simulink model "Safety_filter_obstacle_run_FxTISMC"  (R2022a)
settings: Solver=ode4  StartTime=0.0  StopTime=30  FixedStep=0.01  RelTol=1e-3
libraries: simulink x1
settings Model: PacingRate=0.500000  Creator=14244039  LastModifiedBy=40335991
settings DebuggingCC: UnconnectedInputMsg=warning  UnconnectedOutputMsg=warning  UnconnectedLineMsg=warning  UnderSpecifiedDimensionMsg=warning
settings RTWCC: DLArmComputeVersion=19.05

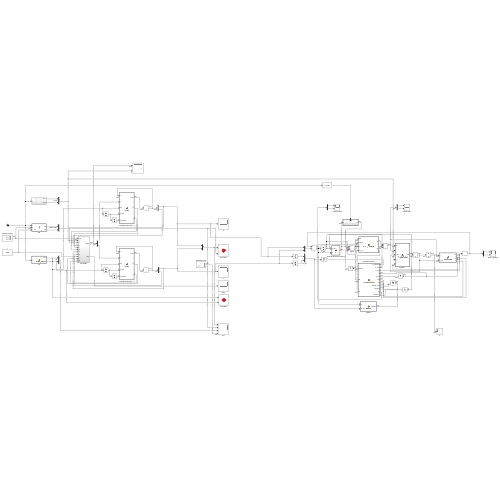
[thumbnail: Simulink's stored preview of the top-level diagram]
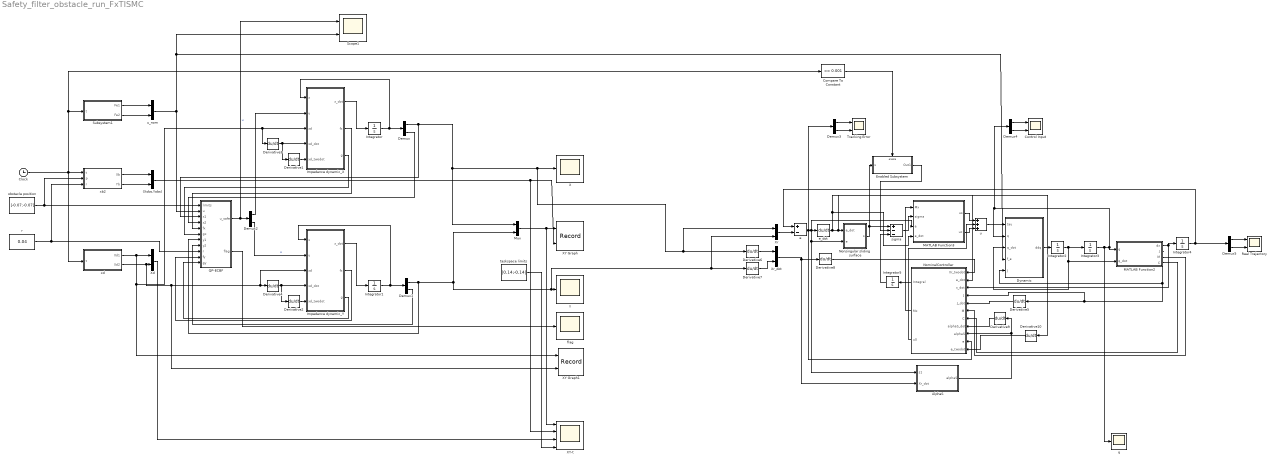
== system Safety_filter_obstacle_run_FxTISMC ==
  " Tracking Error" : Scope  NumInputPorts=2
  (Xobs,Yobs) : Mux  Inputs=2
  AlphaS : MATLAB Function  TreatAsAtomicUnit=on
  Clock : Clock
  Compare To Constant : simulink/Logic and Bit Operations/Compare To Constant  relop=<=  const=0.001  OutDataTypeStr=boolean
  Control Input : Scope  NumInputPorts=2
  Demux{,1..5} (6 alike) : Demux  Outputs=2
  Derivative{1..10} (10 alike) : Derivative
  Dynamic : MATLAB Function  TreatAsAtomicUnit=on
  Enabled Subsystem : Subsystem  TreatAsAtomicUnit=on
  Impedance dynamic_X : MATLAB Function  TreatAsAtomicUnit=on
  Impedance dynamic_Y : MATLAB Function  TreatAsAtomicUnit=on
  Integrator : Integrator  InitialCondition=[0.14;0]
  Integrator1 : Integrator  InitialCondition=[0;0]
  Integrator2 : Integrator
  Integrator3 : Integrator  InitialCondition=[0.5236;2.0944]
  Integrator4 : Integrator  InitialCondition=[0.14;0]
  Integrator5 : Integrator  InitialCondition=[0.0001;0.0001]
  MATLAB Function2 : MATLAB Function  TreatAsAtomicUnit=on
  MATLAB Function3 : MATLAB Function  TreatAsAtomicUnit=on
  Mux : Mux  Inputs=2
  NominalController : MATLAB Function  TreatAsAtomicUnit=on
  Nonsingular sliding surface : MATLAB Function  TreatAsAtomicUnit=on
  QP-ECBF : Subsystem
  Real Trajectory : Scope  NumInputPorts=2
  Scope1 : Scope  NumInputPorts=2
  Subsystem1 : Subsystem
  X : Scope
  XY Graph : Record  FileSettingsInternal="{\"entries\":[{\"content\":{\"excelSettings\":{\"content\":{},\"type\":\"Streamout.ExcelSettings\"}},\"type\":\"Streamout.FileSettingStorage\",\"uuid\":\"41ee0d73-6c9a-4a32-9ae2-bb77aa5eb9da\"}],\"packageUris\":[\"http://schema.mathworks.com/mf0/streamout_blocks/R2020a\"],\"version\":\"1.0\"}"  Layout=[1 1]  SignalsInternal="{\"entries\":[{\"content\":{\"signals\":[{\"content\":{\"blockPath\":[\"Safety_filter_obstacle_run_FxTISMC/XY Graph\"],\"channel\":[],\"dimensions\":[2],\"domain\":\"Safety_filter_obstacle_run_FxTISMC/XY Graph\",\"hasChildren\":true,\"lineColor\":\"#0072bd\",\"plots\":[],\"port\":1,\"sid\":[\"\"],\"signalID\":13917,\"signalName\":\"Mux\"},\"type\":\"RecordBlkView.Signal\",\"uuid\":\"9d963ae4-670a-439a-a92f-b214391dedbc\"},{\"content\":{\"blockPath\":[\"Safety_filter_obstacle_run_FxTISMC/XY Graph\"],\"channel\":[1],\"dimensions\":[2],\"domain\":\"Safety_filter_obstacle_run_FxTISMC/XY Graph\",\"lineColor\":\"#d95319\",\"parentID\":13917,\"plots\":[1],\"port\":1,\"sid\":[\"\"],\"signalID\":13918,\"signalName\":\"Mux\"},\"type\":\"RecordBlkView.Signal\",\"uuid\":\"5de3c74c-0cc7-4e71-b0b3-a53949196780\"},{\"content\":{\"blockPath\":[\"Safety_filter_obstacle_run_FxTISMC/XY Graph\"],\"channel\":[],\"dimensions\":[2],\"domain\":\"Safety_filter_obstacle_run_FxTISMC/XY Graph\",\"hasChildren\":true,\"lineColor\":\"#edb120\",\"plots\":[],\"port\":2,\"sid\":[\"\"],\"signalID\":13922,\"signalName\":\"(Xobs,Yobs)\"},\"type\":\"RecordBlkView.Signal\",\"uuid\":\"3f86d34b-246c-421d-b9f1-6aa0b0fd2e9d\"},{\"content\":{\"blockPath\":[\"Safety_filter_obstacle_run_FxTISMC/XY Graph\"],\"channel\":[1],\"dimensions\":[2],\"domain\":\"Safety_filter_obstacle_run_FxTISMC/XY Graph\",\"lineColor\":\"#7e2f8e\",\"parentID\":13922,\"plots\":[1],\"port\":2,\"sid\":[\"\"],\"signalID\":13923,\"signalName\":\"(Xobs,Yobs)\"},\"type\":\"RecordBlkView.Signal\",\"uuid\":\"b5bee711-287f-47f0-862a-4f60470f5475\"},{\"content\":{\"blockPath\":[\"Safety_filter_obstacle_run_FxTISMC/XY Graph\"],\"channel\":[2],\"dimensions\":[2],\"domain\":\"Safety_filter_obstacle_run_FxTISMC/XY Graph\",\"lineColor\":\"#a2142f\",\"parentID\":13917,\"plots\":[1],\"port\":1,\"sid\":[\"\"],\"signalID\":13935,\"signalName\":\"Mux\"},\"type\":\"RecordBlkView.Signal\",\"uuid\":\"9dfeebbb-1213-4c0a-aa59-e1486d2e2cfe\"},{\"content\":{\"blockPath\":[\"Safety_filter_obstacle_run_FxTISMC/XY Graph\"],\"channel\":[2],\"dimensions\":[2],\"domain\":\"Safety_filter_obstacle_run_FxTISMC/XY Graph\",\"lineColor\":\"#139fff\",\"parentID\":13922,\"plots\":[1],\"port\":2,\"sid\":[\"\"],\"signalID\":13936,\"signalName\":\"(Xobs,Yobs)\"},\"type\":\"RecordBlkView.Signal\",\"uuid\":\"a1ac44f8-5473-466a-96b0-ad1e605dc7af\"}]},\"type\":\"RecordBlkView.InputSignals\",\"uuid\":\"7214ea23-0c5e-4860-8b5d-1e1159aeb053\"}],\"packageUris\":[\"http://schema.mathworks.com/mf0/streamout_blocks/R2020a\"],\"version\":\"1.0\"}"  VisualizationBindings="{\"xyplotplugin\":{\"info\":[{\"series\":[{\"bindingParametersList\":[{\"parameter\":\"X-Axis\",\"signalID\":13918,\"signalName\":\"Mux(1)\"},{\"parameter\":\"Y-Axis\",\"signalID\":13935,\"signalName\":\"Mux(2)\"}],\"seriesID\":62594},{\"bindingParametersList\":[{\"parameter\":\"X-Axis\",\"signalID\":13923,\"signalName\":\"(Xobs,Yobs)(1)\"},{\"parameter\":\"Y-Axis\",\"signalID\":13936,\"signalName\":\"(Xobs,Yobs)(2)\"}],\"seriesID\":13492}],\"subplotID\":1}]}}"  CompatibilityTag=XY  st=-1
  XY Graph1 : Record  FileSettingsInternal="{\"entries\":[{\"content\":{\"excelSettings\":{\"content\":{},\"type\":\"Streamout.ExcelSettings\"}},\"type\":\"Streamout.FileSettingStorage\",\"uuid\":\"947f9a06-cda0-4a39-953d-72ad5f3dd9f2\"}],\"packageUris\":[\"http://schema.mathworks.com/mf0/streamout_blocks/R2020a\"],\"version\":\"1.0\"}"  Layout=[1 1]  SignalsInternal="{\"entries\":[{\"content\":{\"signals\":[{\"content\":{\"blockPath\":[\"Safety_filter_obstacle_run_FxTISMC/XY Graph1\"],\"channel\":[],\"dimensions\":[1],\"domain\":\"Safety_filter_obstacle_run_FxTISMC/XY Graph1\",\"lineColor\":\"#a2142f\",\"plots\":[1],\"port\":1,\"sid\":[\"\"],\"signalID\":13927,\"signalName\":\"xd:1\"},\"type\":\"RecordBlkView.Signal\",\"uuid\":\"bb191c1c-9b05-4e6a-a985-f226d7343dd8\"},{\"content\":{\"blockPath\":[\"Safety_filter_obstacle_run_FxTISMC/XY Graph1\"],\"channel\":[],\"dimensions\":[1],\"domain\":\"Safety_filter_obstacle_run_FxTISMC/XY Graph1\",\"lineColor\":\"#139fff\",\"plots\":[1],\"port\":2,\"sid\":[\"\"],\"signalID\":13931,\"signalName\":\"xd:2\"},\"type\":\"RecordBlkView.Signal\",\"uuid\":\"5ec12a56-9b42-4693-a6cf-ba7cb0d2111f\"}]},\"type\":\"RecordBlkView.InputSignals\",\"uuid\":\"53783b2f-f43d-4ce0-a107-2c856c2899e0\"}],\"packageUris\":[\"http://schema.mathworks.com/mf0/streamout_blocks/R2020a\"],\"version\":\"1.0\"}"  VisualizationBindings="{\"xyplotplugin\":{\"info\":[{\"series\":[{\"bindingParametersList\":[{\"parameter\":\"X-Axis\",\"signalID\":13927,\"signalName\":\"xd:1\"},{\"parameter\":\"Y-Axis\",\"signalID\":13931,\"signalName\":\"xd:2\"}],\"seriesID\":52353}],\"subplotID\":1}]}}"  CompatibilityTag=XY
  XY-t : Scope  NumInputPorts=4
  Xd : Mux  Inputs=2
  Xr : Mux  Inputs=2
  Xr_dot : Mux  Inputs=2
  Y : Scope
  e : Sum  Inputs=+-
  e_dot : Derivative
  flag : Scope
  obstacle position : Constant  Value=[-0.07;-0.07]  VectorParams1D=off  SampleTime=-1
  q : Scope
  r : Constant  Value=0.04  VectorParams1D=off  SampleTime=-1
  sigma : Sum  Inputs=+--
  taskspace limits : Constant  Value=[0.14;-0.14]  VectorParams1D=off  SampleTime=-1
  u : Sum  Inputs=+++
  u_nom : Mux  Inputs=2
  xb2 : MATLAB Function  TreatAsAtomicUnit=on
  xd : MATLAB Function  TreatAsAtomicUnit=on
  wires:
  Subsystem1/1(Fe1) -> u_nom/1
  Clock/1 -> Compare To Constant/1, Subsystem1/1(t), xd/1(t), xb2/1(t)
  Derivative3/1 -> Impedance dynamic_X/4(xd_dot), Derivative1/1
  Derivative1/1 -> Impedance dynamic_X/5(xd_twodot)
  Impedance dynamic_X/1(x_dot) -> Integrator/1
  Integrator/1 -> Demux/1, Impedance dynamic_X/1(x)
  Demux2/2 -> Impedance dynamic_Y/2(u)  "u"
  xd/2(Xd2) -> XY Graph1/2, Impedance dynamic_Y/3(xd), Derivative4/1, Xd/2
  Impedance dynamic_Y/1(x_dot) -> Integrator1/1
  Derivative4/1 -> Impedance dynamic_Y/4(xd_dot), Derivative2/1
  Derivative2/1 -> Impedance dynamic_Y/5(xd_twodot)
  Integrator1/1 -> Demux1/1, Impedance dynamic_Y/1(x)
  Subsystem1/2(Fe2) -> u_nom/2
  xb2/1(Xb) -> (Xobs,Yobs)/1
  xb2/2(Yb) -> (Xobs,Yobs)/2
  Mux/1 -> XY-t/1, XY Graph/1
  (Xobs,Yobs)/1 -> XY-t/2, XY Graph/2
  QP-ECBF/1(u_safe) -> Scope1/1, Demux2/1  "u"
  Demux2/1 -> Impedance dynamic_X/2(u)
  obstacle position/1 -> QP-ECBF/1(limits), xb2/2(p)
  Demux/2 -> QP-ECBF/4(x2)
  Impedance dynamic_X/2(fx) -> QP-ECBF/5(fx)
  Impedance dynamic_X/3(g) -> QP-ECBF/6(gx)
  Demux1/2 -> QP-ECBF/8(y2)
  r/1 -> xb2/3(r), QP-ECBF/9(r)
  QP-ECBF/2(flag) -> flag/1
  Impedance dynamic_Y/2(fx) -> QP-ECBF/10(fy)
  Impedance dynamic_Y/3(g) -> QP-ECBF/11(gy)
  xd/1(Xd1) -> XY Graph1/1, Impedance dynamic_X/3(xd), Derivative3/1, Xd/1
  Xd/1 -> XY-t/3
  taskspace limits/1 -> XY-t/4
  NominalController/1(Integral) -> Integrator5/1
  Demux5/2 -> Real Trajectory/2
  Demux4/2 -> Control Input/2
  Integrator5/1 -> sigma/3
  u_nom/1 -> Dynamic/4(f_e), Scope1/2, QP-ECBF/2(u)
  e_dot/1 -> MATLAB Function3/4(e_dot), Derivative10/1, NominalController/2(e_dot), Nonsingular sliding surface/1(e_dot)
  Nonsingular sliding surface/1(s) -> Enabled Subsystem/1(s), sigma/1
  Demux4/1 -> Control Input/1
  AlphaS/1(alphaS) -> Derivative9/1, NominalController/9(alphaS)
  Enabled Subsystem/1(Out1) -> sigma/2
  Demux3/2 -> " Tracking Error"/2
  Dynamic/1(ddq) -> Integrator2/1
  Demux3/1 -> " Tracking Error"/1
  Xr/1 -> e/2
  Compare To Constant/1 -> Enabled Subsystem/Enable
  MATLAB Function2/4(C) -> NominalController/7(C)
  Derivative9/1 -> NominalController/8(alphaS_dot)
  MATLAB Function3/1(us) -> u/1
  MATLAB Function2/1(dx) -> Integrator4/1, NominalController/3(x_dot)
  MATLAB Function3/2(uc) -> u/3
  Derivative10/1 -> NominalController/11(e_twodot)
  Derivative8/1 -> NominalController/1(Xr_twodot)
  u/1 -> Dynamic/1(tau)
  MATLAB Function2/2(J) -> Dynamic/5(J), NominalController/4(J), Derivative5/1
  Integrator3/1 -> q/1, Demux4/1, Dynamic/2(q), MATLAB Function2/1(q)
  Xr_dot/1 -> AlphaS/2(Xr_dot), Derivative8/1
  sigma/1 -> MATLAB Function3/2(sigma)
  Integrator4/1 -> Demux5/1, e/1
  MATLAB Function2/3(M) -> NominalController/6(M)
  e/1 -> Demux3/1, e_dot/1, MATLAB Function3/3(e), AlphaS/1(s1), Nonsingular sliding surface/2(e), NominalController/10(e)
  NominalController/2(Mx) -> MATLAB Function3/1(Mx)
  Integrator2/1 -> MATLAB Function2/2(q_dot), Dynamic/3(q_dot), Integrator3/1
  NominalController/3(u0) -> u/2
  Demux5/1 -> Real Trajectory/1
  Derivative5/1 -> NominalController/5(J_dot)
  Demux1/1 -> QP-ECBF/7(y1), Xr/2, Derivative7/1, Y/1, Mux/2
  Demux/1 -> QP-ECBF/3(x1), Mux/1, Xr/1, Derivative6/1, X/1
  Derivative6/1 -> Xr_dot/1
  Derivative7/1 -> Xr_dot/2

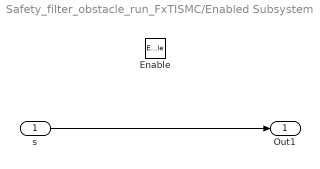
== system Safety_filter_obstacle_run_FxTISMC/Enabled Subsystem ==
  s : Inport
  Enable : EnablePort
  Out1 : Outport  InitialOutput=0  VectorParamsAs1DForOutWhenUnconnected=off
  wires:
  s/1 -> Out1/1

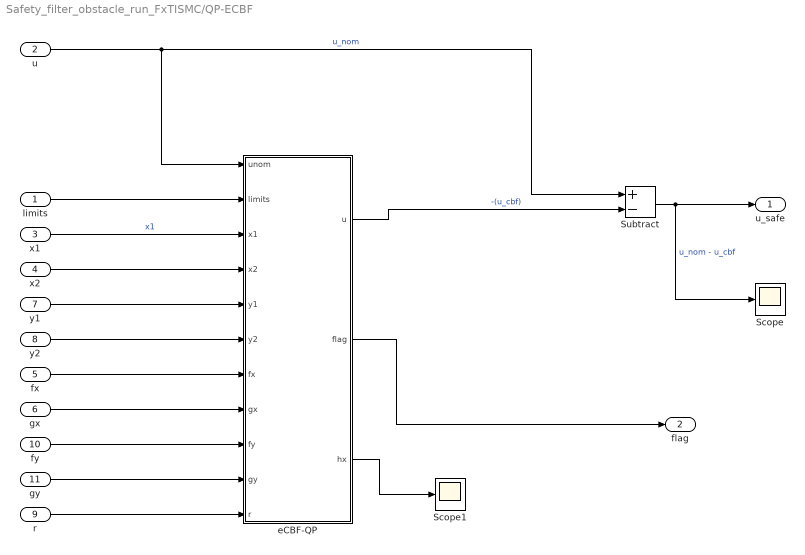
== system Safety_filter_obstacle_run_FxTISMC/QP-ECBF ==
  limits : Inport
  u : Inport  Port=2
  x1 : Inport  Port=3
  x2 : Inport  Port=4
  fx : Inport  Port=5
  gx : Inport  Port=6
  y1 : Inport  Port=7
  y2 : Inport  Port=8
  r : Inport  Port=9
  fy : Inport  Port=10
  gy : Inport  Port=11
  Scope : Scope
  Scope1 : Scope
  Subtract : Sum  Inputs=+-
  eCBF-QP : MATLAB Function  TreatAsAtomicUnit=on
  u_safe : Outport
  flag : Outport  Port=2
  wires:
  x2/1 -> eCBF-QP/4(x2)
  limits/1 -> eCBF-QP/2(limits)
  u/1 -> eCBF-QP/1(unom), Subtract/1  "u_nom"
  x1/1 -> eCBF-QP/3(x1)  "x1"
  eCBF-QP/1(u) -> Subtract/2  "-(u_cbf)"
  Subtract/1 -> u_safe/1, Scope/1  "u_nom - u_cbf"
  fx/1 -> eCBF-QP/7(fx)
  gx/1 -> eCBF-QP/8(gx)
  eCBF-QP/2(flag) -> flag/1
  y1/1 -> eCBF-QP/5(y1)
  y2/1 -> eCBF-QP/6(y2)
  r/1 -> eCBF-QP/11(r)
  eCBF-QP/3(hx) -> Scope1/1
  fy/1 -> eCBF-QP/9(fy)
  gy/1 -> eCBF-QP/10(gy)

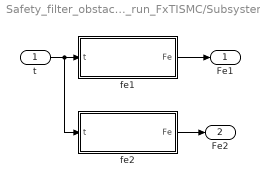
== system Safety_filter_obstacle_run_FxTISMC/Subsystem1 ==
  t : Inport
  fe1 : MATLAB Function  TreatAsAtomicUnit=on
  fe2 : MATLAB Function  TreatAsAtomicUnit=on
  Fe1 : Outport
  Fe2 : Outport  Port=2
  wires:
  fe1/1(Fe) -> Fe1/1
  fe2/1(Fe) -> Fe2/1
  t/1 -> fe2/1(t), fe1/1(t)

== matlab function Safety_filter_obstacle_run_FxTISMC/MATLAB Function2 ==
  data: q input; q_dot input; dx output; J output; M output; C output
function [dx,J,M,C]  = JointTwoTask(q,q_dot)
L = [0.3, 0.3];
m = [1.5, 1];

M = [m(2)*L(2)^2+2*m(2)*L(1)*L(2)*cos(q(2))+(m(1)+m(2))*L(1)^2, m(2)*L(2)^2+m(2)*L(1)*L(2)*cos(q(2));
    m(2)*L(2)^2+m(2)*L(1)*L(2)*cos(q(2)), m(2)*L(2)^2];
C = [-2*m(2)*L(1)*L(2)*sin(q(2))*q_dot(2), -m(2)*L(1)*L(2)*sin(q(2)); 
    m(2)*L(1)*L(2)*sin(q(2))*q_dot(1), 0];
J = [-L(1)*sin(q(1))-L(2)*sin(q(1)+q(2)), -L(2)*sin(q(1)+q(2));
    L(1)*cos(q(1))+L(2)*cos(q(1)+q(2)), L(2)*cos(q(1)+q(2))];
dx = J*q_dot;
end

== matlab function Safety_filter_obstacle_run_FxTISMC/AlphaS ==
  data: s1 input; alphaS output; Xr_dot input
function alphaS = AlphaS(s1,Xr_dot)

k1=3;
k2=20;
k3=50;

alpha=5/7;
beta=5/3;

alphaS = -(k1.*s1 + k2.*abs(s1).^alpha.*sign(s1) + k3.*abs(s1).^beta.*sign(s1)) + Xr_dot;

end

== matlab function Safety_filter_obstacle_run_FxTISMC/MATLAB Function3 ==
  data: Mx input; us output; sigma input; uc output; e input; e_dot input
function [us,uc] = ISMC_Controller(Mx,sigma,e,e_dot)

K_gain=0.001;
k1=20;
k2=50;
alpha=5/3;
beta=5/7;
Mxx=pinv(Mx);
gamma = 5/7;
us = -inv(Mx)*((K_gain+0.001)*sign(sigma) + k1*abs(sigma).^alpha.*sign(sigma) + k2*abs(sigma).^beta.*sign(sigma));
% uc = -Mxx*k2^gamma*(abs(e_dot+k1*abs(e).^alpha.*sign(e)).^(1/gamma-1)).*e_dot;
uc = 0;
end

== matlab function Safety_filter_obstacle_run_FxTISMC/NominalController ==
  data: Xr_twodot input; e_dot input; x_dot input size=[2 1]; J input; J_dot input; M input; C input; alphaS_dot input size=[2 1]; Integral output size=[2 1]; Mx output size=[2 2]; u0 output size=[2 1]; alphaS input; e input; e_twodot input
function [Integral,Mx,u0] = NominalController(Xr_twodot,e_dot,x_dot,J,J_dot,M,C,alphaS_dot,alphaS,e,e_twodot)

Mx = inv(J')*M*inv(J);
Cx = inv(J')*(C-(M*inv(J)*J_dot))*inv(J);

%% PD Controller
% Kp=35;
% Kd=400;
% f=Mx*(Kp*(Xr-x)+Kd*(Xr_dot-x_dot)) + Cx*x_dot;
% u0=(J')*f;

%% Fixed-time backstepping control
k8=3;
k9=20;
k10=50;
alpha=5/3;
beta=5/7;
gamma = 5/7;

s2 = x_dot - alphaS;

f0 = Mx*(inv(Mx)*Cx*x_dot + alphaS_dot - k8*s2 - k9*abs(s2).^alpha.*sign(s2) - k10*abs(s2).^beta.*sign(s2));
u0=(J')*f0;

%% Integral term of fixed-time integral sliding mode controller

k1=20;
k2=50;
%  Integral = Mx\u0 +  Mx\Cx*x_dot - Xr_twodot + e_dot + (1/k2^gamma)*(abs(e_dot+k1*abs(e).^alpha.*sign(e)).^(1/gamma-1)).*(Mx\u0 +  Mx\Cx*x_dot - Xr_twodot + k1*abs(e).^(alpha-1).*e_dot);
Integral = e_dot + (1/k2^gamma)*(abs(e_dot+k1*abs(e).^alpha.*sign(e)).^(1/gamma-1)).*(Mx\u0 +  Mx\Cx*x_dot - Xr_twodot + k1*abs(e).^(alpha-1).*e_dot);


end

== matlab function Safety_filter_obstacle_run_FxTISMC/Nonsingular sliding surface ==
  data: e_dot input; e input; s output
function s = S(e_dot,e)

k1=20;
k2=50;
alpha=5/3;
beta=5/7;
gamma = 5/7;

s = e + (1/k2^(gamma)).*abs(e_dot+k1*abs(e).^alpha.*sign(e)).^(1/gamma).*sign(e_dot+k1*abs(e).^alpha.*sign(e));

end

== matlab function Safety_filter_obstacle_run_FxTISMC/xb2 ==
  data: t input; Xb output; Yb output; p input; r input
function [Xb,Yb]  = Obstacles_traj(t,p,r)

Xb =  p(1) + r*cos(t);
Yb =  p(2) + r*sin(t);
    
end

== matlab function Safety_filter_obstacle_run_FxTISMC/Impedance dynamic_Y ==
  data: x input size=[2 1]; u input; x_dot output size=[2 1]; xd input; xd_dot input; xd_twodot input; fx output; g output
function [x_dot,fx,g] = System(x,u,xd,xd_dot,xd_twodot)

    km = 20;
    kb = 20;                                                       
    kk = 100;
    fx = [x(2);
        -(1/km)*(kb*(x(2)-xd_dot)+kk*(x(1)-xd)-km*xd_twodot)];
    g = [0;km^(-1)];
    x_dot = fx + g*u;
end

== matlab function Safety_filter_obstacle_run_FxTISMC/Subsystem1/fe1 ==
  data: t input; Fe output
function Fe  = External_force(t)

   Fe = 0*(t<4|t>=11) + (1-cos(pi*t))*(t>=4&t<5) + 2*(t>=5&t<10) + (1+cos(pi*t))*(t>=10&t<11);

end

== matlab function Safety_filter_obstacle_run_FxTISMC/Dynamic ==
  data: tau input size=[2 1]; ddq output size=[2 1]; q input size=[2 1]; q_dot input size=[2 1]; f_e input; J input
function ddq  = TwoLinkRobot(tau,q,q_dot,f_e,J)
L = [0.3, 0.3];
m = [1.5, 1];
g = 9.8;

M = [m(2)*L(2)^2+2*m(2)*L(1)*L(2)*cos(q(2))+(m(1)+m(2))*L(1)^2, m(2)*L(2)^2+m(2)*L(1)*L(2)*cos(q(2));
    m(2)*L(2)^2+m(2)*L(1)*L(2)*cos(q(2)), m(2)*L(2)^2];
C = [-2*m(2)*L(1)*L(2)*sin(q(2))*q_dot(2), -m(2)*L(1)*L(2)*sin(q(2)); 
    m(2)*L(1)*L(2)*sin(q(2))*q_dot(1), 0];

F=[2*cos(q(1))*sin(q(2))+5*cos(q(1))^2;-2*cos(q(1))*sin(q(2))-5*cos(q(1))^2];

tau_e = (J')*f_e;
ddq = M\(-C*q_dot-F + tau + tau_e);

end

== matlab function Safety_filter_obstacle_run_FxTISMC/Subsystem1/fe2 ==
  data: t input; Fe output
function Fe  = External_force(t)

   Fe = 0*(t<4|t>=11) + 2*(1-cos(pi*t))*(t>=4&t<5) + 4*(t>=5&t<10) + 2*(1+cos(pi*t))*(t>=10&t<11);

end

== matlab function Safety_filter_obstacle_run_FxTISMC/xd ==
  data: t input; Xd1 output; Xd2 output
function [Xd1, Xd2] = Desired_traj(t)

    Xd1=0.14*cos(0.5*t);
    Xd2=0.14*sin(0.5*t);
    
end

== matlab function Safety_filter_obstacle_run_FxTISMC/QP-ECBF/eCBF-QP ==
  settings: updateMethod=DISCRETE
  data: unom input; limits input; u output size=[2 1]; x1 input; x2 input; y1 input; y2 input; fx input; gx input; fy input; gy input; flag output; r input; hx output
function [u,flag,hx] = fcn(unom, limits, x1, x2,y1 ,y2 ,fx,gx,fy,gy,r)
    %% Obstacle position
    X_obs    = limits(1);
    Y_obs    = limits(2);
    fe_x = unom(1);
    fe_y = unom(2);
    %% ECBF Gains
    k1 = 70;
    k2 = 700;
    r = r+0.01;
    %% CBF 
    hx      = (x1 - X_obs)^2 + (y1 - Y_obs)^2 - r^2 ; 
    Lfhx    = 2*(x1 - X_obs)*x2 + 2*(y1 - Y_obs)*y2;
    L2fhx_unom = 2*(x1 - X_obs)*( gx(2)*fe_x) + 2*(y1 - Y_obs)*( gy(2)*fe_y) ;

    L2fhx_usafe_x = 2*(x1 - X_obs)*gx(2);
    L2fhx_usafe_y = 2*(y1 - Y_obs)*gy(2);
   

    H       = [2 0; 0 2];
    f       = [0;0]; 
    
    A       = [L2fhx_usafe_x, L2fhx_usafe_y]; 
            
    b       = [L2fhx_unom + k1*Lfhx + k2*hx];
    X   = [0;0];
    flag = 0;
    coder.extrinsic('quadprog');
    [output, ~, flag]   = quadprog(H,f,A,b,[],[],[],[]);

    if flag == 1
        X = output;
    else
        X   = [0;0];
    end
    
%Function outputs
    u = X; 
end

== matlab function Safety_filter_obstacle_run_FxTISMC/Impedance dynamic_X ==
  data: x input size=[2 1]; u input; x_dot output size=[2 1]; xd input; xd_dot input; xd_twodot input; fx output; g output
function [x_dot,fx,g] = System(x,u,xd,xd_dot,xd_twodot)

    km = 20;
    kb = 20;                                                       
    kk = 100;
    fx = [x(2);
        -(1/km)*(kb*(x(2)-xd_dot)+kk*(x(1)-xd)-km*xd_twodot)];
    g = [0;km^(-1)];
    x_dot = fx + g*u;
end
